simulink model "mathmodel"  (R2022b)
settings: Solver=VariableStepAuto  StartTime=0.0  StopTime=10.0  RelTol=1e-3
values from neighbouring files (symbols this model uses):
  U = [U_n,U_p]    [UI.m]
undefined symbols (not defined in the file or in its folder): J, ke, Km, L, R
settings Model: Creator=tameembourgi  LastModifiedBy=tameembourgi

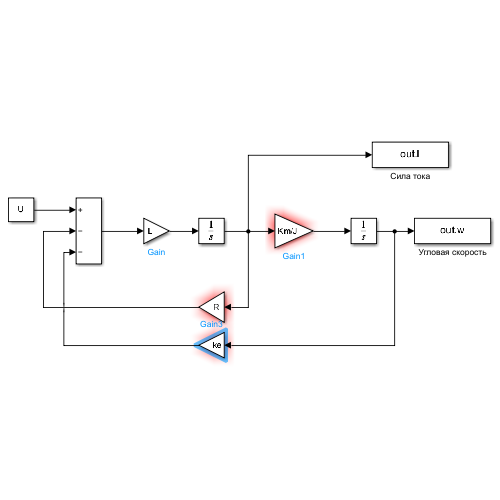
[thumbnail: Simulink's stored preview of the top-level diagram]
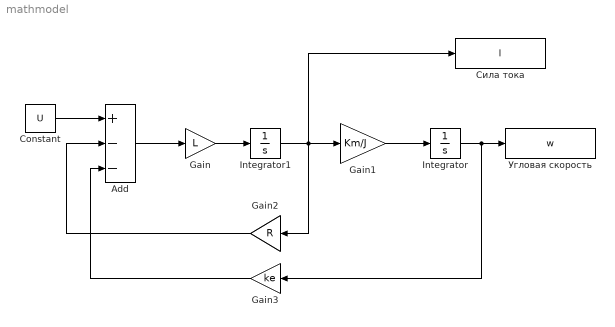
== system mathmodel ==
  Add : Sum  Inputs=+--
  Constant : Constant  Value=U
  Gain : Gain  Gain=L
  Gain1 : Gain  Gain=Km/J
  Gain2 : Gain  Gain=R
  Gain3 : Gain  Gain=ke
  Integrator : Integrator
  Integrator1 : Integrator
  Сила тока : ToWorkspace  VariableName=l  SaveFormat=Timeseries  SampleTime=-1
  Угловая скорость : ToWorkspace  VariableName=w  SaveFormat=Timeseries  SampleTime=-1
  wires:
  Constant/1 -> Add/1
  Add/1 -> Gain/1
  Gain/1 -> Integrator1/1
  Integrator1/1 -> Сила тока/1, Gain2/1, Gain1/1
  Gain1/1 -> Integrator/1
  Integrator/1 -> Gain3/1, Угловая скорость/1
  Gain3/1 -> Add/3
  Gain2/1 -> Add/2
